simulink model "ImpedanceControl"  (R2014a)
settings: Solver=FixedStepAuto  StartTime=0.0  StopTime=10.0  FixedStep=Ts  RelTol=1e-3  EnableMultiTasking=on
settings Model: Creator=faezeh  LastModifiedBy=faezeh
settings DataIOCC: LimitDataPoints=off
settings OptimizationCC: SimCompilerOptimization=off
settings DebuggingCC: MergeDetectMultiDrivingBlocksExec=error  FcnCallInpInsideContextMsg=error  FrameProcessingCompatibilityMsg=error  SFExecutionAtInitializationDiag=none  ArithmeticOperatorsInVariantConditions=warning
settings HardwareCC: ProdBitPerSizeT=32  ProdBitPerPtrDiffT=32
settings RTWCC: RTWCompilerOptimization=off
settings CodeAppCC: StateflowObjectComments=on
settings ConfigComp: CovMetricSettings=dw  CovHtmlReporting=on  CovSaveCumulativeToWorkspaceVar=on  CovSaveSingleToWorkspaceVar=on  CovExternalEMLEnable=off  CovSFcnEnable=off

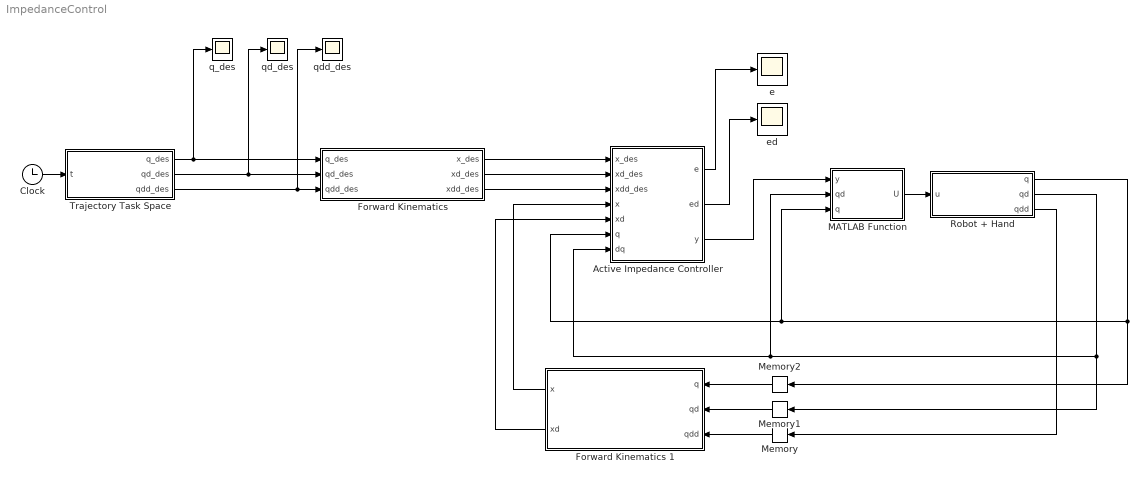
== system ImpedanceControl ==
  Active Impedance Controller : MATLAB Function  TreatAsAtomicUnit=on
  Clock : Clock
  "Forward Kinematics " : MATLAB Function  TreatAsAtomicUnit=on
  Forward Kinematics 1 : MATLAB Function  TreatAsAtomicUnit=on
  MATLAB Function : MATLAB Function  TreatAsAtomicUnit=on
  Memory : Memory
  Memory1 : Memory
  Memory2 : Memory
  "Robot + Hand " : Subsystem
  Trajectory Task Space : MATLAB Function  TreatAsAtomicUnit=on
  e : Scope
  ed : Scope
  q_des : Scope
  qd_des : Scope
  qdd_des : Scope
  wires:
  Clock/1 -> Trajectory Task Space/1(t)
  Trajectory Task Space/1(q_des) -> "Forward Kinematics "/1(q_des), q_des/1
  Trajectory Task Space/2(qd_des) -> "Forward Kinematics "/2(qd_des), qd_des/1
  Trajectory Task Space/3(qdd_des) -> "Forward Kinematics "/3(qdd_des), qdd_des/1
  "Forward Kinematics "/1(x_des) -> Active Impedance Controller/1(x_des)
  "Forward Kinematics "/2(xd_des) -> Active Impedance Controller/2(xd_des)
  Active Impedance Controller/3(y) -> MATLAB Function/1(y)
  MATLAB Function/1(U) -> "Robot + Hand "/1("u ")
  "Robot + Hand "/1(q) -> Memory2/1, Active Impedance Controller/6(q), MATLAB Function/3(q)
  "Forward Kinematics "/3(xdd_des) -> Active Impedance Controller/3(xdd_des)
  Active Impedance Controller/1(e) -> e/1
  Active Impedance Controller/2(ed) -> ed/1
  "Robot + Hand "/2(qd) -> Memory1/1, Active Impedance Controller/7(dq), MATLAB Function/2(qd)
  "Robot + Hand "/3(qdd) -> Memory/1
  Forward Kinematics 1/1(x) -> Active Impedance Controller/4(x)
  Forward Kinematics 1/2(xd) -> Active Impedance Controller/5(xd)
  Memory/1 -> Forward Kinematics 1/3(qdd)
  Memory1/1 -> Forward Kinematics 1/2(qd)
  Memory2/1 -> Forward Kinematics 1/1(q)

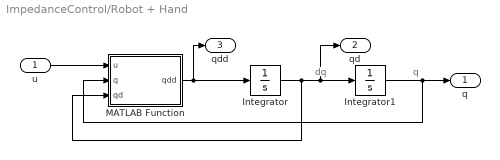
== system ImpedanceControl/Robot + Hand  ==
  note: q
  note: dq
  "u " : Inport  PortDimensions=3
  Integrator : Integrator  InitialCondition=[0;0;0]
  Integrator1 : Integrator  InitialCondition=[0;0;0]
  MATLAB Function : MATLAB Function  TreatAsAtomicUnit=on
  q : Outport  PortDimensions=3
  qd : Outport  Port=2  PortDimensions=3
  qdd : Outport  Port=3  PortDimensions=3
  wires:
  "u "/1 -> MATLAB Function/1(u)
  MATLAB Function/1(qdd) -> qdd/1, Integrator/1
  Integrator/1 -> MATLAB Function/3(qd), qd/1, Integrator1/1
  Integrator1/1 -> MATLAB Function/2(q), q/1

== matlab function ImpedanceControl/Active Impedance Controller ==
  data: e output; ed output; x_des input; y output; xd_des input; xdd_des input; x input; xd input; q input; dq input
function [e,ed,y] = ImpController(x_des,xd_des,xdd_des,x,xd,q,dq)
    %% Recalling Model Kinematics
    q1=q(1);q2=q(2);q3=q(3);
    dq1=dq(1);dq2=dq(2);dq3=dq(3);
   [~,J,Jd] = KinematicModel(q1,q2,q3,dq1,dq2,dq3);
    %% Impedance Behaviour Parameters
    Md =100*eye(6);       % Interia matrix, must be Positive definite
    Kd =500*eye(6);       % Damping matrix
    Kp =2500*eye(6);       % stiffness matrix
    
    %% Error Calculation
    %task error
    e = x_des-x;
    ed = xd_des-xd;

    %% Impedance Input
    y = pinv(J)*inv(Md)*(Md*xdd_des + Kd*ed + Kp*e - Md*Jd*dq);

end

== matlab function ImpedanceControl/Forward Kinematics  ==
  data: q_des input; x_des output; qd_des input; xd_des output; xdd_des output; qdd_des input
function [x_des,xd_des,xdd_des]  = ForwardKinematics(q_des,qd_des,qdd_des)
q1=q_des(1);q2=q_des(2);q3=q_des(3);
dq1=qd_des(1);dq2=qd_des(2);dq3=qd_des(3);
[Te,j,jd] = KinematicModel(q1,q2,q3,dq1,dq2,dq3);
p=Te(1:3,4);
R7=Te(1:3,1:3);
f=atan2(R7(2,1),R7(1,1));
t=atan2(-R7(3,1),sqrt(R7(3,2)^2+R7(3,3)^2));
s=atan2(R7(3,2),R7(3,3)); 
RPY=[s;t;f]; %R7PY R7epR7esentation
% f=atan2(R7(2,1),R7(1,1));
% t=atan2(-R7(3,1),sqrt(R7(3,2)^2+R7(3,3)^2));
% s=atan2(R7(3,2),R7(3,3));
% euler=[f;t;s];
x_des = [p;RPY];
xd_des = j*qd_des;
xdd_des = jd*qd_des + j*qdd_des;

== matlab function ImpedanceControl/Robot + Hand /MATLAB Function ==
  data: u input; qdd output; q input; qd input
function qdd = DirDyn(u,q,qd)
%% Recalling Model Dynamics 
[M,V,G] = DynamicModel(q,qd);
B=[0.0252; 0.0019; 0.0029]; %Nms/rad
Fk=[0.1891; 0.0541; 0.1339];
Jmeta=35.9*0.9*0.9*[1;1;1]*0.001*0.0001;
M=M+[Jmeta(1) 0 0;0 Jmeta(2) 0;0 0 Jmeta(3)]; 
he=[0;0;0;0;0;0];
%% Recalling Model Dynamics 
q1=q(1);q2=q(2);q3=q(3);
dq1=qd(1);dq2=qd(2);dq3=qd(3);
[~,J,~] = KinematicModel(q1,q2,q3,dq1,dq2,dq3);
qdd =inv(M)*(u -(V + G + B.*qd + Fk.*sign(qd) + J.'*he ));

== matlab function ImpedanceControl/Trajectory Task Space ==
  data: t input; q_des output; qd_des output; qdd_des output
function [q_des,qd_des,qdd_des]       = TRJ(t)
   %% trapezoidal velocity profile 
   qf=[30;10;10];
   qf=qf*(pi/180);
   qi=[0;0;0];
   L=norm(qf-qi);
   qd_max=0.1; %v_max enterd by user
   T=100*qd_max;
   qdd_max=qd_max^2/(T*qd_max-L);
   sig=0;
   sigd=0;
   sigdd=0;

   Ts=qd_max/qdd_max;
   if t<=Ts
   sig=qdd_max*t^2/2;
   sigd=qdd_max*t;
   sigdd=qdd_max;
   elseif t>Ts && t<=(T-Ts)
   sig=qd_max*t-(qd_max)^2/(2*qdd_max);
   sigd=qd_max;
   sigdd=0;
   elseif t>(T-Ts) && t<=T
   sig=-qdd_max*(t-T)^2/2+qd_max*T-(qd_max)^2/qdd_max;
   sigd=-qdd_max*(t-T);
   sigdd=-qdd_max;
   end

   %% Line Trajecory 
   q_des = qi + sig*(qf-qi)/L;
   qd_des = (qf-qi)*sigd/L;
   qdd_des = (qf-qi)*sigdd/L;
end

== matlab function ImpedanceControl/Forward Kinematics 1 ==
  data: q input; x output; qd input; xd output; qdd input
function [x,xd]  = ForwardKinematics(q,qd,qdd)
q1=q(1);q2=q(2);q3=q(3);
dq1=qd(1);dq2=qd(2);dq3=qd(3);
[Te,j,jd] = KinematicModel(q1,q2,q3,dq1,dq2,dq3);
p=Te(1:3,4);
R7=Te(1:3,1:3);
f=atan2(R7(2,1),R7(1,1));
t=atan2(-R7(3,1),sqrt(R7(3,2)^2+R7(3,3)^2));
s=atan2(R7(3,2),R7(3,3)); 
RPY=[s;t;f]; %R7PY R7epR7esentation
% f=atan2(R7(2,1),R7(1,1));
% t=atan2(-R7(3,1),sqrt(R7(3,2)^2+R7(3,3)^2));
% s=atan2(R7(3,2),R7(3,3));
% euler=[f;t;s];
x = [p;RPY];
xd = j*qd;

== matlab function ImpedanceControl/MATLAB Function ==
  data: y input; U output; qd input; q input
function U = Controller(y,qd,q)   
    %% Recalling Model Dynamics 
    [M,V,G] = DynamicModel(q,qd);
    B=[0.0252; 0.0019; 0.0029]; %Nms/rad
    Fk=[0.1891; 0.0541; 0.1339]; %Nm
    Jmeta=35.9*0.9*0.9*[1;1;1]*0.001*0.0001;
    M=M+[Jmeta(1) 0 0;0 Jmeta(2) 0;0 0 Jmeta(3)]; 
    %% Controller Command
     U = M*y + V + G + B.*qd + Fk.*sign(qd);
end
